simulink model "anim_tp_comde_NL"  (R2019b)
settings: Solver=ode5  StartTime=0  StopTime=12  FixedStep=.005  MaxStep=0.02  RelTol=1e-3  AbsTol=1e-6
values from neighbouring files (symbols this model uses):
  g = 9.8    [cobs.m]
  L = 1    [cobs.m]
  M = 5    [cobs.m]
  m = 0.5    [cobs.m]
settings Model: Creator=user  LastModifiedBy=user
settings SolverCC: AutoScaleAbsTol=off
settings DataIOCC: ExternalInput=[]  InitialState=[]  SaveFormat=Array  SignalLoggingSaveFormat=ModelDataLogs  SaveOutput=off  SaveTime=off  ReturnWorkspaceOutputs=off
settings OptimizationCC: BooleanDataType=off  ExpressionDepthLimit=2147483647  InitFltsAndDblsToZero=on  LifeSpan=inf
settings DebuggingCC: SaveWithParameterizedLinksMsg=none  UnderspecifiedInitializationDetection=Classic  MergeDetectMultiDrivingBlocksExec=none  SignalResolutionControl=TryResolveAllWithWarning  MultiTaskDSMMsg=warning  MultiTaskCondExecSysMsg=none  FcnCallInpInsideContextMsg=warning  StateNameClashWarn=warning  SFUnexpectedBacktrackingDiag=warning  SFNoUnconditionalDefaultTransitionDiag=warning  SFExecutionAtInitializationDiag=none  ArithmeticOperatorsInVariantConditions=warning
settings HardwareCC: ProdBitPerPointer=32  ProdBitPerSizeT=32  ProdBitPerPtrDiffT=32  ProdLargestAtomicFloat=None  ProdIntDivRoundTo=Undefined  ProdEndianess=Unspecified  ProdWordSize=32  ProdHWDeviceType=32-bit Generic  TargetUnknown=on
settings ModelReferenceCC: PropagateSignalLabelsOutOfModel=off
settings SFSimCC: SimUseLocalCustomCode=off  CustomCodeUndefinedFunction=UseInterfaceOnly
settings RTWCC: RTWUseLocalCustomCode=off
settings CodeAppCC: StateflowObjectComments=on
settings GRTTargetCC: TargetFcnLib=ansi_tfl_tmw.mat  TargetLangStandard=C89/C90 (ANSI)  GeneratePreprocessorConditionals=Disable all  CombineOutputUpdateFcns=off  GRTInterface=on
settings ConfigComp: CovMetricSettings=dw  CovHtmlReporting=on  CovSaveCumulativeToWorkspaceVar=on  CovSaveSingleToWorkspaceVar=on  CovExternalEMLEnable=off

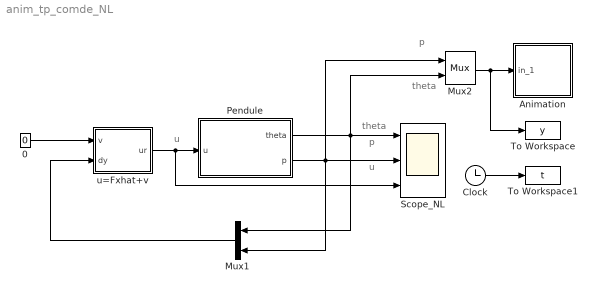
== system anim_tp_comde_NL ==
  note: theta
  note: p
  note: theta
  note: p
  note: u
  note: u
  0 : Constant  Value=0
  Animation : Subsystem  mask(Animation du déplacement du pendule inverse){}
      mask Help: Fonction d'animation du pendule inverse (voir s_fonction tp_pendan_g.m.
      mask Display: plot([-10 10],[0 0],[-2 -2 2 2],[0 1 1 0],[0 -3],[1 5])
  Clock : Clock
  Mux1 : Mux  Inputs=2
  Mux2 : Mux  Inputs=2
  Pendule : Subsystem  mask(Pendule inverse sur un chariot (éq. Non Linéaires)){M=M, m=m, l=L, g=g, x0=[0.1 0 0.1 0]}
      mask prompts: M "Masse du chariot (kg):"; m "Masse du pendule (kg):"; l "Longueur de la barre (m):"; g "gravité (m/s^2):"; x0 "Conditions Initiales [theta theta' p p']"
      mask help: Utiliser le menu "Look under mask" pour voir les équations de la dynamique (celles de l'énoncé du TP)
      mask Help: Description Non Linéaire de la dynamique d'un pendule inverse sur un chariot.
      mask Display:
      | plot([-10 10],[1 1],[-2 -2 2 2],[1 2 2 1],[0 3],[2 5])
      | text(-13,0.5,'Eq. Non Linéaires')
      | plot([-14 14],[-0.5 -0.5])
  Scope_NL : Scope  NumInputPorts=3
  To Workspace : ToWorkspace  VariableName=y  SampleTime=0.1
  To Workspace1 : ToWorkspace  VariableName=t  SampleTime=0.1
  u=Fxhat+v : Subsystem
  wires:
  Mux2/1 -> To Workspace/1, Animation/1(in_1)
  Clock/1 -> To Workspace1/1
  u=Fxhat+v/1(ur) -> Pendule/1(u), Scope_NL/3
  Mux1/1 -> u=Fxhat+v/2(dy)
  0/1 -> u=Fxhat+v/1(v)
  Pendule/2(p) -> Mux1/2, Mux2/1, Scope_NL/2
  Pendule/1(theta) -> Mux1/1, Mux2/2, Scope_NL/1

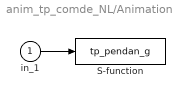
== system anim_tp_comde_NL/Animation ==
  in_1 : Inport
  S-function : S-Function  FunctionName=tp_pendan_g  SFunctionDeploymentMode=off  EnableBusSupport=off
      settings: DeleteFcn=pendan([],[],[],'DeleteBlock');
  wires:
  in_1/1 -> S-function/1

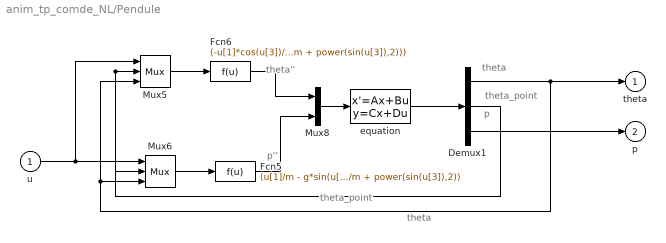
== system anim_tp_comde_NL/Pendule ==
  note: theta
  note: theta_point
  note: p''
  note: theta''
  note: theta
  note: theta_point
  note: p
  u : Inport
  Demux1 : Demux  Outputs=3
  Fcn5 : Fcn  Expr=(u[1]/m - g*sin(u[3])*cos(u[3]) + l*power(u[2],2)*sin(u[3]))/(M/m + power(sin(u[3]),2))
  Fcn6 : Fcn  Expr=(-u[1]*cos(u[3])/m + (M+m)*g*sin(u[3])/m - l*power(u[2],2)*sin(u[3])*cos(u[3]))/(l*(M/m + power(sin(u[3]),2)))
  Mux5 : Mux  Inputs=3
  Mux6 : Mux  Inputs=3
  Mux8 : Mux  Inputs=2
  equation : StateSpace  A=[ 0 1 0 0 ; 0 0 0 0 ; 0 0 0 1; 0 0 0 0]  B=[0 0 ; 1 0 ; 0 0 ; 0 1]  C=[1 0 0 0 ; 0 1 0 0 ; 0 0 1 0]  D=zeros(3,2)  InitialCondition=x0
  theta : Outport  InitialOutput=0
  p : Outport  Port=2  InitialOutput=0
  wires:
  u/1 -> Mux6/1, Mux5/1
  Mux6/1 -> Fcn5/1
  Mux5/1 -> Fcn6/1
  Demux1/2 -> Mux5/2, Mux6/2
  equation/1 -> Demux1/1
  Fcn6/1 -> Mux8/1
  Fcn5/1 -> Mux8/2
  Mux8/1 -> equation/1
  Demux1/1 -> Mux6/3, Mux5/3, theta/1
  Demux1/3 -> p/1

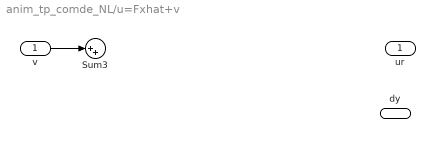
== system anim_tp_comde_NL/u=Fxhat+v ==
  v : Inport
  dy : Inport  Port=2
  Sum3 : Sum  Inputs=|++  SaturateOnIntegerOverflow=on  InputSameDT=on  OutDataTypeStr=Inherit: Same as first input
  ur : Outport
  wires:
  v/1 -> Sum3/1
